simulink model "PTC_MBDS_StringConcat_Sample"  (R2013a)
settings: Solver=FixedStepDiscrete  StartTime=0.0  StopTime=100  FixedStep=0.02  RelTol=1e-3
libraries: PTC_MBDS_LIB x7, simulink_extras x1
settings Model: BufferReuse=off  Creator=sundeep.tuteja  LastModifiedBy=sundeep.tuteja
settings OptimizationCC: BlockReduction=off  OptimizeBlockIOStorage=off  BufferReuse=off  ExpressionFolding=off  LocalBlockOutputs=off
settings HardwareCC: ProdIntDivRoundTo=Zero  ProdEndianess=LittleEndian  ProdHWDeviceType=Generic->Custom  TargetIntDivRoundTo=Zero  TargetEndianess=LittleEndian  TargetHWDeviceType=Generic->Custom
settings RTWCC: ProcessScript=grt_make_rtw_hook

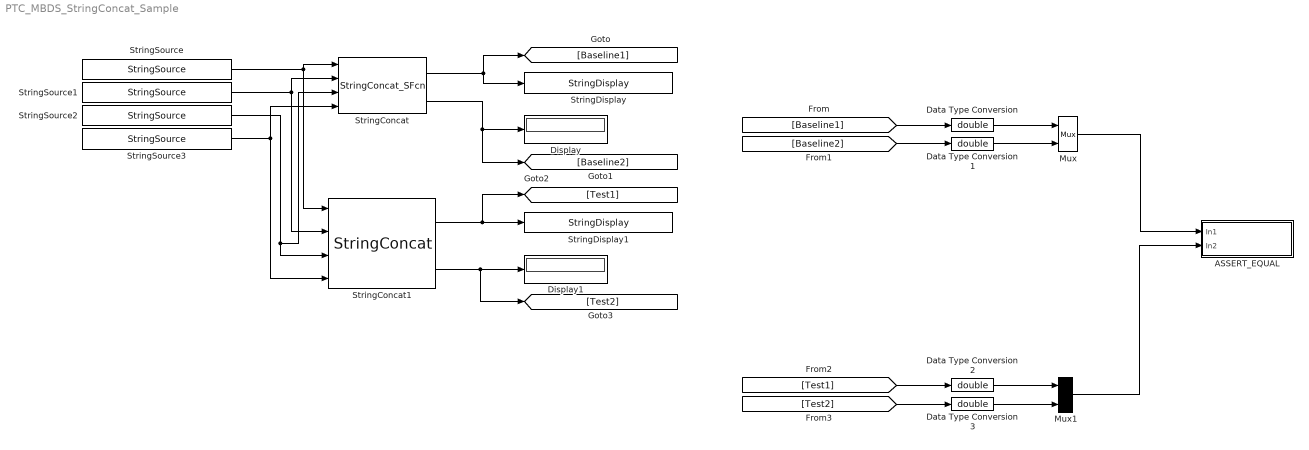
== system PTC_MBDS_StringConcat_Sample ==
  ASSERT_EQUAL : Subsystem
  Data Type Conversion{,1..3} (4 alike) : DataTypeConversion  OutDataTypeStr=double
  Display : Display
  Display1 : Display
  Mux : Mux  Inputs=2
  Mux1 : Mux  Inputs=2
  StringConcat : S-Function  InitFcn=|  FunctionName=StringConcat_SFcn  Parameters=boolean(ENO_Enabled), uint16(StringNumber), uint16(MaxStringLength)  EnableBusSupport=off  mask(StringConcat){MBDS_LibraryBlock=on, ENO_Enabled=on, StringNumber=4, MBDS_BlockVersion=05.40}
      | if(exist('MBDS_BlockCallback', 'file'))
      |    MBDS_BlockCallback('Update', gcb);
      | end
      mask prompts: MBDS_LibraryBlock "MBDS Library Block"; ENO_Enabled "Show ENO port"; StringNumber "Number of inputs (min. 2, max. 10):"; MBDS_BlockVersion "Block version:"
      mask help: Concatenates all input strings to one string. The resulting string length is limited to the maximum string length defined by the project options.
      mask init:
      | MBDS_BlockCallback('Copy', gcb);
      | MaxStringLength = 1 + GetStringLen();
      | maskdisplay = ['disp(''Concat'')' 10];
      | if(~isnumeric(StringNumber) || StringNumber < 2)
      |    StringNumber = 2;
      | end
      | if(StringNumber > 10)
      |    StringNumber = 10;
      | end
      | for k = [1:StringNumber]
      |    maskdisplay = [maskdisplay 'port_label(''input'', ' num2str(k) ', ''In' num2str(k) ''')' 10];
      | end
      | maskdisplay = [maskdisplay 'port_label(''output'', 1, ''Out'')' 10];
      | if(ENO_Enabled)
      | 	maskdisplay = [maskdisplay 'port_label(''output'', 2, ''ENO'')' 10];
      | end
      | set_param(gcbh, 'maskdisplay', maskdisplay)
      | UpdateBlockSize(gcb);
      mask Help: eval(['open([workdir(''Library_Dir:''),''\Blockset\Help\'',get_param(gcb,''MaskType''),''.html''])'])
      mask Callback StringNumber:
      | StringNumber = str2double(get_param(gcb, 'StringNumber'));
      | if(StringNumber < 2)
      |    set_param(gcb, 'StringNumber', '2');
      | elseif(StringNumber > 10)
      |    set_param(gcb, 'StringNumber', '10');
      | end
      | clear StringNumber;
      mask Display:
      | disp('Concat')
      | port_label('input', 1, 'In1')
      | port_label('input', 2, 'In2')
      | port_label('input', 3, 'In3')
      | port_label('input', 4, 'In4')
      | port_label('output', 1, 'Out')
      | port_label('output', 2, 'ENO')
  StringConcat1 : PTC_MBDS_LIB/MBDS Standard Library/Extended Operations/String Operations/StringConcat  ENO_Enabled=on  StringNumber=4  MaxStringLength=PTC_MBDS_MaxStringLength_Fcn  PTC_MBDS_BlockVersion=5.32  PTC_BlockType=PTC_MBDS_StringConcat
  StringDisplay : PTC_MBDS_LIB/MBDS Standard Library/Extended Operations/String Operations/StringDisplay  MaxRowCount=1  BlockSignature=----------  PTC_MBDS_BlockVersion=5.32  PTC_BlockType=PTC_MBDS_StringDisplay  DisplayString=MyString000000000000MyStringMyStringMyStr  MaxStringLength=PTC_MBDS_MaxStringLength_Fcn
  StringDisplay1 : PTC_MBDS_LIB/MBDS Standard Library/Extended Operations/String Operations/StringDisplay  MaxRowCount=1  BlockSignature=----------  PTC_MBDS_BlockVersion=5.32  PTC_BlockType=PTC_MBDS_StringDisplay  DisplayString=MyString000000000000MyStringMyStringMyStr  MaxStringLength=PTC_MBDS_MaxStringLength_Fcn
  StringSource : PTC_MBDS_LIB/MBDS Standard Library/Extended Operations/String Operations/StringSource  InputValue=MyString000000000000  PTC_MBDS_BlockVersion=5.32  PTC_BlockType=PTC_MBDS_StringSource  Value=uint8([77; 121; 83; 116; 114; 105; 110; 103; 48; 48; 48; 48; 48; 48; 48; 48; 48; 48; 48; 48; 0; 0; 0; 0; 0; 0; 0; 0; 0; 0; 0; 0; 0; 0; 0; 0; 0; 0; 0; 0; 0])  MaxStringLength=PTC_MBDS_MaxStringLength_Fcn
  StringSource1 : PTC_MBDS_LIB/MBDS Standard Library/Extended Operations/String Operations/StringSource  InputValue=MyString  PTC_MBDS_BlockVersion=5.32  PTC_BlockType=PTC_MBDS_StringSource  Value=uint8([77; 121; 83; 116; 114; 105; 110; 103; 0; 0; 0; 0; 0; 0; 0; 0; 0; 0; 0; 0; 0; 0; 0; 0; 0; 0; 0; 0; 0; 0; 0; 0; 0; 0; 0; 0; 0; 0; 0; 0; 0])  MaxStringLength=PTC_MBDS_MaxStringLength_Fcn
  StringSource2 : PTC_MBDS_LIB/MBDS Standard Library/Extended Operations/String Operations/StringSource  InputValue=MyString  PTC_MBDS_BlockVersion=5.32  PTC_BlockType=PTC_MBDS_StringSource  Value=uint8([77; 121; 83; 116; 114; 105; 110; 103; 0; 0; 0; 0; 0; 0; 0; 0; 0; 0; 0; 0; 0; 0; 0; 0; 0; 0; 0; 0; 0; 0; 0; 0; 0; 0; 0; 0; 0; 0; 0; 0; 0])  MaxStringLength=PTC_MBDS_MaxStringLength_Fcn
  StringSource3 : PTC_MBDS_LIB/MBDS Standard Library/Extended Operations/String Operations/StringSource  InputValue=MyString  PTC_MBDS_BlockVersion=5.32  PTC_BlockType=PTC_MBDS_StringSource  Value=uint8([77; 121; 83; 116; 114; 105; 110; 103; 0; 0; 0; 0; 0; 0; 0; 0; 0; 0; 0; 0; 0; 0; 0; 0; 0; 0; 0; 0; 0; 0; 0; 0; 0; 0; 0; 0; 0; 0; 0; 0; 0])  MaxStringLength=PTC_MBDS_MaxStringLength_Fcn
  wires:
  Mux1/1 -> ASSERT_EQUAL/2(In2)
  Mux/1 -> ASSERT_EQUAL/1(In1)
  Data Type Conversion/1 -> Mux/1
  Data Type Conversion1/1 -> Mux/2
  Data Type Conversion2/1 -> Mux1/1
  Data Type Conversion3/1 -> Mux1/2
  StringSource/1 -> StringConcat/1, StringConcat1/1
  StringSource1/1 -> StringConcat/2, StringConcat1/2
  StringSource2/1 -> StringConcat/3, StringConcat1/3
  StringSource3/1 -> StringConcat/4, StringConcat1/4
  StringConcat/2 -> [Baseline2], Display/1
  StringConcat1/2 -> [Test2], Display1/1
  StringConcat/1 -> StringDisplay/1, [Baseline1]
  StringConcat1/1 -> [Test1], StringDisplay1/1
  [Baseline1] -> Data Type Conversion/1
  [Baseline2] -> Data Type Conversion1/1
  [Test1] -> Data Type Conversion2/1
  [Test2] -> Data Type Conversion3/1

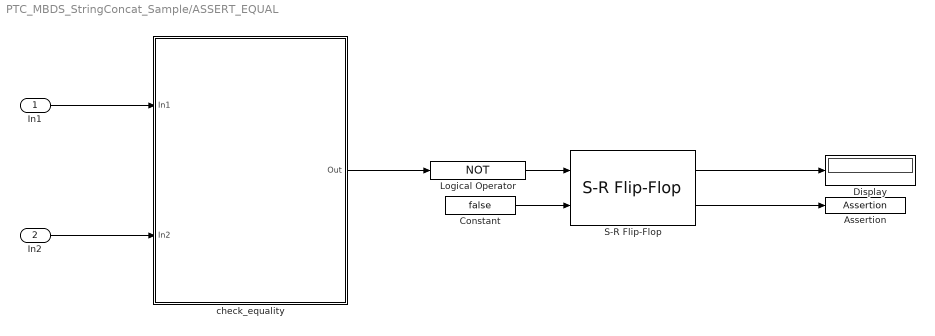
== system PTC_MBDS_StringConcat_Sample/ASSERT_EQUAL ==
  In1 : Inport
  In2 : Inport  Port=2
  Assertion : Assertion
  Constant : Constant  Value=false
  Display : Display
  Logical Operator : Logic  Operator=NOT  AllPortsSameDT=off  OutDataTypeStr=boolean
  S-R Flip-Flop : simulink_extras/Flip Flops/S-R Flip-Flop  initial_condition=0
  check_equality : MATLAB Function  TreatAsAtomicUnit=on
  wires:
  S-R Flip-Flop/1 -> Display/1
  check_equality/1(Out) -> Logical Operator/1
  Constant/1 -> S-R Flip-Flop/2
  S-R Flip-Flop/2 -> Assertion/1
  In2/1 -> check_equality/2(In2)
  In1/1 -> check_equality/1(In1)
  Logical Operator/1 -> S-R Flip-Flop/1

== matlab function PTC_MBDS_StringConcat_Sample/ASSERT_EQUAL/check_equality ==
  data: In1 input; Out output; In2 input
function Out = check_equality(In1, In2)
%#codegen

Out = isequaln(In1, In2);

end
